simulink library "MinSegLibrary_M1V4"  (R2015a)
settings: Solver=ode45  StartTime=0.0  StopTime=10.0  RelTol=1e-3
libraries: arduinolib x8
settings Model: Creator=hurstj  LastModifiedBy=008399924
settings DebuggingCC: UnderspecifiedInitializationDetection=Classic  MergeDetectMultiDrivingBlocksExec=none  SolverPrmCheckMsg=warning  StateNameClashWarn=warning

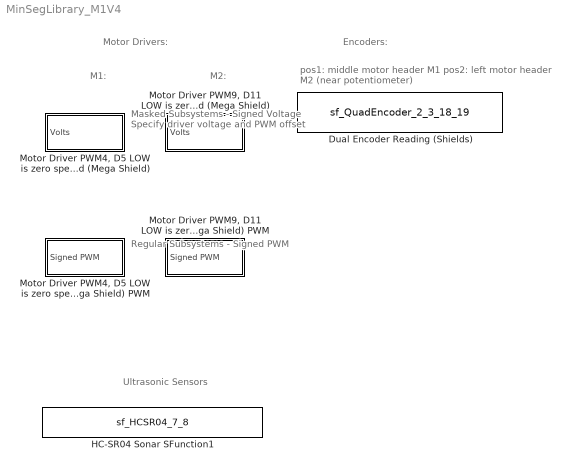
== system MinSegLibrary_M1V4 ==
  note: M1:
  note: Masked Subsystems - Signed Voltage
      | Specify driver voltage and PWM offset
  note: Motor Drivers:
  note: Encoders:
  note: Ultrasonic Sensors
  note: Regular Subsystems - Signed PWM
  note: pos1: middle motor header M1
      | pos2: left motor header M2 (near potentiometer)
  note: M2:
  Dual Encoder Reading (Shields) : S-Function  InitFcn=try, set_param(gcb,'FunctionName','sf_QuadEncoder_2_3_18_19'), end  FunctionName=sf_QuadEncoder_2_3_18_19  Parameters=uint8([0 1]),uint8([2 18]),uint8([3 19])  SFunctionModules=sf_QuadEncoder_2_3_18_19_wrapper  mask(S-Function Builder){}
      mask init:
      | val = [[.9  0.75 0.75 1 1 .9 .9 1]',[1 1 0.75 0.75 .9 .9 1 .9]'];try , sys = get_param(gcb,'SfunBuilderFcnName');if isempty(sys), sys = get_param(gcb,'FunctionName'); end,catch, sys = get_param(gcb,'FunctionName'); end
      settings: CopyFcn=set_param(gcbh,'LinkStatus','none')  PreSaveFcn=try, set_param(gcb,'FunctionName','sf_QuadEncoder_2_3_18_19'), end  OpenFcn=sfunctionwizard(gcbh)
      mask Display: plot(val(:,1),val(:,2)),disp(sys), port_label('output',1,'pos1'), port_label('output',2,'pos2')
  HC-SR04 Sonar SFunction1 : S-Function  InitFcn=try, set_param(gcb,'FunctionName','sf_HCSR04_7_8'), end  FunctionName=sf_HCSR04_7_8  SFunctionModules=sf_HCSR04_7_8_wrapper  mask(S-Function Builder){}
      mask help: Simulink:masks:SFunctionBuilder_MD
      mask init: same as MinSegLibrary_M1V4/Dual Encoder Reading (Shields)
      settings: CopyFcn=set_param(gcbh,'LinkStatus','none')  PreSaveFcn=try, set_param(gcb,'FunctionName','sf_HCSR04_7_8'), end  OpenFcn=sfunctionwizard(gcbh)
      mask Display:
      | plot(val(:,1),val(:,2))
      | disp(sys)
      | port_label('output',1,'distance_cm')
  "Motor Driver PWM4, D5 LOW is zero speed (Mega Shield)" : Subsystem  mask{Vsupply=4.5, PWMoffset=0}
      mask prompts: Vsupply "Driver Voltage"; PWMoffset "PWM offset (0-255)"
      mask help:
      | Specify driver supply voltage (4.5 for USB)
      | Specify the PWM offset (0-255)
  "Motor Driver PWM4, D5 LOW is zero speed (Mega Shield) PWM" : Subsystem
  "Motor Driver PWM9, D11 LOW is zero speed (Mega Shield)" : Subsystem  mask{Vsupply=4.5, PWMoffset=0}
      mask prompts: Vsupply "Driver Voltage"; PWMoffset "PWM offset (0-255)"
      mask help:
      | Specify driver supply voltage (4.5 for USB)
      | Specify the PWM offset (0-255)
  "Motor Driver PWM9, D11 LOW is zero speed (Mega Shield) PWM" : Subsystem

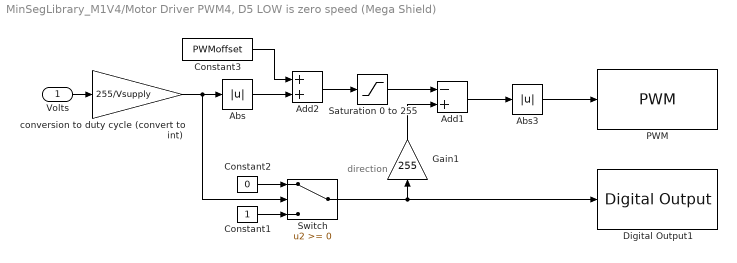
== system MinSegLibrary_M1V4/Motor Driver PWM4, D5 LOW is zero speed (Mega Shield) ==
  note: direction
  Volts : Inport
  Abs : Abs
  Abs3 : Abs
  Add1 : Sum  Inputs=-+
  Add2 : Sum
  Constant1 : Constant
  Constant2 : Constant  Value=0
  Constant3 : Constant  Value=PWMoffset
  Digital Output1 : arduinolib/Digital Output  pinNumber=5
  Gain1 : Gain  Gain=255
  PWM : arduinolib/PWM  pinNumber=4
  Saturation 0 to 255 : Saturate  UpperLimit=255  LowerLimit=0
  Switch : Switch
  conversion to duty cycle (convert to int) : Gain  Gain=255/Vsupply  OutDataTypeStr=int16
  wires:
  Volts/1 -> conversion to duty cycle (convert to int)/1
  Switch/1 -> Digital Output1/1, Gain1/1
  Constant2/1 -> Switch/1
  Constant1/1 -> Switch/3
  Gain1/1 -> Add1/2
  Add1/1 -> Abs3/1
  conversion to duty cycle (convert to int)/1 -> Switch/2, Abs/1
  Saturation 0 to 255/1 -> Add1/1
  Abs3/1 -> PWM/1
  Constant3/1 -> Add2/1
  Abs/1 -> Add2/2
  Add2/1 -> Saturation 0 to 255/1

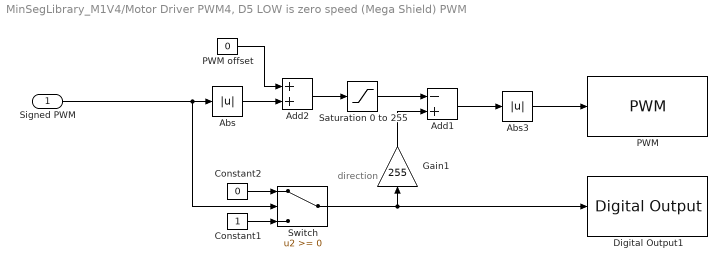
== system MinSegLibrary_M1V4/Motor Driver PWM4, D5 LOW is zero speed (Mega Shield) PWM ==
  note: direction
  Signed PWM : Inport
  Abs : Abs
  Abs3 : Abs
  Add1 : Sum  Inputs=-+
  Add2 : Sum
  Constant1 : Constant
  Constant2 : Constant  Value=0
  Digital Output1 : arduinolib/Digital Output  pinNumber=5
  Gain1 : Gain  Gain=255
  PWM : arduinolib/PWM  pinNumber=4
  PWM offset : Constant  Value=0
  Saturation 0 to 255 : Saturate  UpperLimit=255  LowerLimit=0
  Switch : Switch
  wires:
  Switch/1 -> Digital Output1/1, Gain1/1
  Constant2/1 -> Switch/1
  Constant1/1 -> Switch/3
  Gain1/1 -> Add1/2
  Add1/1 -> Abs3/1
  Signed PWM/1 -> Switch/2, Abs/1
  Saturation 0 to 255/1 -> Add1/1
  Abs3/1 -> PWM/1
  PWM offset/1 -> Add2/1
  Abs/1 -> Add2/2
  Add2/1 -> Saturation 0 to 255/1

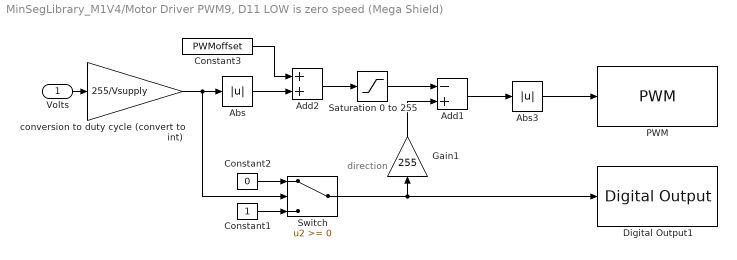
== system MinSegLibrary_M1V4/Motor Driver PWM9, D11 LOW is zero speed (Mega Shield) ==
  note: direction
  Volts : Inport
  Abs : Abs
  Abs3 : Abs
  Add1 : Sum  Inputs=-+
  Add2 : Sum
  Constant1 : Constant
  Constant2 : Constant  Value=0
  Constant3 : Constant  Value=PWMoffset
  Digital Output1 : arduinolib/Digital Output  pinNumber=11
  Gain1 : Gain  Gain=255
  PWM : arduinolib/PWM  pinNumber=9
  Saturation 0 to 255 : Saturate  UpperLimit=255  LowerLimit=0
  Switch : Switch
  conversion to duty cycle (convert to int) : Gain  Gain=255/Vsupply  OutDataTypeStr=int16
  wires:
  Add2/1 -> Saturation 0 to 255/1
  Abs/1 -> Add2/2
  Constant3/1 -> Add2/1
  Abs3/1 -> PWM/1
  Saturation 0 to 255/1 -> Add1/1
  conversion to duty cycle (convert to int)/1 -> Abs/1, Switch/2
  Add1/1 -> Abs3/1
  Gain1/1 -> Add1/2
  Constant1/1 -> Switch/3
  Constant2/1 -> Switch/1
  Switch/1 -> Gain1/1, Digital Output1/1
  Volts/1 -> conversion to duty cycle (convert to int)/1

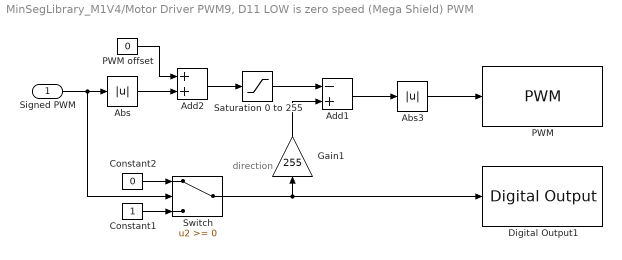
== system MinSegLibrary_M1V4/Motor Driver PWM9, D11 LOW is zero speed (Mega Shield) PWM ==
  note: direction
  Signed PWM : Inport
  Abs : Abs
  Abs3 : Abs
  Add1 : Sum  Inputs=-+
  Add2 : Sum
  Constant1 : Constant
  Constant2 : Constant  Value=0
  Digital Output1 : arduinolib/Digital Output  pinNumber=11
  Gain1 : Gain  Gain=255
  PWM : arduinolib/PWM  pinNumber=9
  PWM offset : Constant  Value=0
  Saturation 0 to 255 : Saturate  UpperLimit=255  LowerLimit=0
  Switch : Switch
  wires:
  Switch/1 -> Digital Output1/1, Gain1/1
  Constant2/1 -> Switch/1
  Constant1/1 -> Switch/3
  Gain1/1 -> Add1/2
  Add1/1 -> Abs3/1
  Signed PWM/1 -> Switch/2, Abs/1
  Saturation 0 to 255/1 -> Add1/1
  Abs3/1 -> PWM/1
  PWM offset/1 -> Add2/1
  Abs/1 -> Add2/2
  Add2/1 -> Saturation 0 to 255/1
